simulink model "PID_ControlSim"  (R2018a)
settings: Solver=VariableStepAuto  StartTime=0.0  StopTime=10  FixedStep=0.01  MaxStep=0.01  RelTol=1e-3
values from neighbouring files (symbols this model uses):
  b = 0.5*mp*Lp*Lr*Bp    [InvPend_PID.m]
  b2 = -0.5*mp*Lp*Lr*Bp / JT    [InvPend_PID.m]
  c = 0.25*mp^2*Lp^2*Lr*gty    [InvPend_PID.m]    (also in InvPend_Params.m = 0.0318)
  c2 = 0.25*mp^2*Lp^2*Lr*gty / JT    [InvPend_PID.m]
  d = ( Jp + 0.25*mp*Lp^2 ) * ( etag*etam*kt/Rm )    [InvPend_PID.m]    (also in InvPend_Params.m = 0.1522)
  d2 = ( Jp + 0.25*mp*Lp^2 )*( etag*etam*kt )/( JT*Rm )    [InvPend_PID.m]
  f = ( Jr + mp*Lr^2 )*Bp    [InvPend_PID.m]
  g = 0.5*mp*Lp*gty*( Jr + mp*Lr^2 )    [InvPend_PID.m]
  g2 = -( Jr + mp*Lr^2 )*Bp / JT    [InvPend_PID.m]
  h = ( 0.5*mp*Lp*Lr ) * ( etag*etam*kt/Rm )    [InvPend_PID.m]
  h2 = 0.5*mp*Lp*gty*( Jr + mp*Lr^2 ) / JT    [InvPend_PID.m]
  i2 = ( 0.5*mp*Lp*Lr )*( etag*etam*kt )/( JT*Rm )    [InvPend_PID.m]
  JT = Jp*mp*Lr^2 + Jr*Jp + 0.25*Jr*mp*Lp^2    (= 2.04748555487e-06)    [InvPend_Params.m]
  Kd = K    (= 0.465)    [InvPend_PID.m]
  Ki = zc1*zc2*K    [InvPend_PID.m]
  Kp = (zc1 + zc2)*K    [InvPend_PID.m]
  q = a + d*Kg*km    [InvPend_PID.m]
  q2 = g2 + a2 + e2    [InvPend_PID.m]
  r = e + h*Kg*km    [InvPend_PID.m]    (also in InvPend_StateSpace.m = 0.35*square(0.1*2*pi*t))
  r2 = -h2 + g2*( a2 + e2 ) - b2*( f2 + j2 )    [InvPend_PID.m]
  t2 = h2*( a2 + e2 ) - c2*( f2 + j2 )    [InvPend_PID.m]
libraries: simulink_extras x2, simulink x1
settings Model: Creator=andrewchulock  LastModifiedBy=andrewchulock

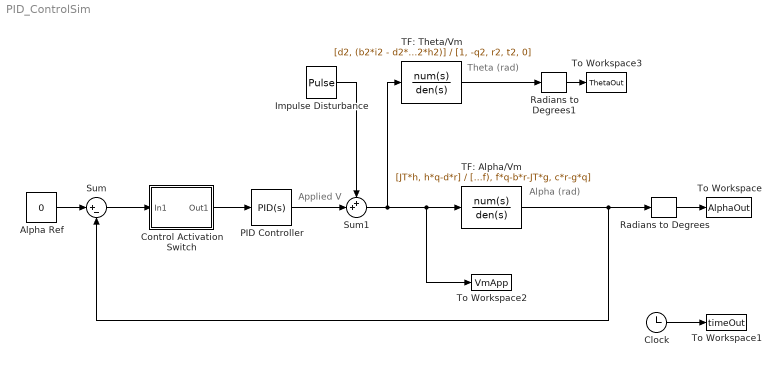
== system PID_ControlSim ==
  note: Theta (rad)
  note: Applied V
  note: Alpha (rad)
  Alpha Ref : Constant  Value=0
  Clock : Clock
  Control Activation Switch : Subsystem
  Impulse Disturbance : DiscretePulseGenerator  PulseType=Time based  Period=10  PulseWidth=0.01  PhaseDelay=1
  PID Controller : simulink/Continuous/PID Controller  Controller=PID  TimeDomain=Continuous-time  SampleTime=-1  IntegratorMethod=Forward Euler  FilterMethod=Forward Euler  Form=Parallel  UseFilter=on  ControllerParametersSource=internal  P=Kp  I=Ki  D=Kd  N=1  InitialConditionSource=internal  InitialConditionForIntegrator=0  InitialConditionForFilter=0  ExternalReset=none  LimitOutput=off  UpperSaturationLimit=inf  LowerSaturationLimit=-inf  LinearizeAsGain=on  AntiWindupMode=none  Kb=1  TrackingMode=off  Kt=1  PParamMin=[]  PParamMax=[]  IParamMin=[]  IParamMax=[]  DParamMin=[]  DParamMax=[]  NParamMin=[]  NParamMax=[]  KbParamMin=[]  KbParamMax=[]  KtParamMin=[]  KtParamMax=[]  POutMin=[]  POutMax=[]  IOutMin=[]  IOutMax=[]  DOutMin=[]  DOutMax=[]  NOutMin=[]  NOutMax=[]  KbOutMin=[]  KbOutMax=[]  KtOutMin=[]  KtOutMax=[]  IntegratorOutMin=[]  IntegratorOutMax=[]  FilterOutMin=[]  FilterOutMax=[]  SumOutMin=[]  SumOutMax=[]  SumI1OutMin=[]  SumI1OutMax=[]  SumI2OutMin=[]  SumI2OutMax=[]  SumI3OutMin=[]  SumI3OutMax=[]  SumDOutMin=[]  SumDOutMax=[]  SaturationOutMin=[]  SaturationOutMax=[]  IntegratorContinuousStateAttributes=''  IntegratorStateMustResolveToSignalObject=off  IntegratorRTWStateStorageClass=Auto  FilterContinuousStateAttributes=''  FilterStateMustResolveToSignalObject=off  FilterRTWStateStorageClass=Auto  DifferentiatorICPrevScaledInput=0  DifferentiatorOutMin=[]  DifferentiatorOutMax=[]  FilterDiffOutCoefMin=[]  FilterDiffOutCoefMax=[]  SumDenOutMin=[]  SumDenOutMax=[]  SumNumOutMin=[]  SumNumOutMax=[]  ReciprocalOutMin=[]  ReciprocalOutMax=[]  DivideOutMin=[]  DivideOutMax=[]  TunerSelectOption=Transfer Function Based (PID Tuner App)
  Radians to Degrees : simulink_extras/Transformations/Radians to Degrees
  Radians to Degrees1 : simulink_extras/Transformations/Radians to Degrees
  Sum : Sum  Inputs=|+-
  Sum1 : Sum  Inputs=++|
  TF: Alpha/Vm : TransferFcn  Numerator=[JT*h, h*q-d*r]  Denominator=[JT^2, JT*(q+f), f*q-b*r-JT*g, c*r-g*q]
  TF: Theta/Vm : TransferFcn  Numerator=[d2, (b2*i2 - d2*g2), (c2*i2 - d2*h2)]  Denominator=[1, -q2, r2, t2, 0]
  To Workspace : ToWorkspace  VariableName=AlphaOut  SampleTime=-1
      settings: Save2DSignal=2-D array (concatenate along first dimension)
  To Workspace1 : ToWorkspace  VariableName=timeOut  SampleTime=-1
      settings: Save2DSignal=2-D array (concatenate along first dimension)
  To Workspace2 : ToWorkspace  VariableName=VmApp  SampleTime=-1
      settings: Save2DSignal=2-D array (concatenate along first dimension)
  To Workspace3 : ToWorkspace  VariableName=ThetaOut  SampleTime=-1
      settings: Save2DSignal=2-D array (concatenate along first dimension)
  wires:
  TF: Alpha/Vm/1 -> Radians to Degrees/1, Sum/2
  Clock/1 -> To Workspace1/1
  Alpha Ref/1 -> Sum/1
  Control Activation Switch/1(Out1) -> PID Controller/1
  Sum/1 -> Control Activation Switch/1(In1)
  PID Controller/1 -> Sum1/2
  Sum1/1 -> TF: Theta/Vm/1, To Workspace2/1, TF: Alpha/Vm/1
  Impulse Disturbance/1 -> Sum1/1
  TF: Theta/Vm/1 -> Radians to Degrees1/1
  Radians to Degrees/1 -> To Workspace/1
  Radians to Degrees1/1 -> To Workspace3/1

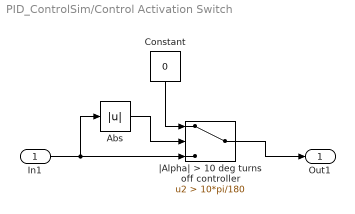
== system PID_ControlSim/Control Activation Switch ==
  In1 : Inport
  " |Alpha| > 10 deg turns off controller" : Switch  Criteria=u2 > Threshold  Threshold=10*pi/180
  Abs : Abs
  Constant : Constant  Value=0
  Out1 : Outport
  wires:
  Constant/1 -> " |Alpha| > 10 deg turns off controller"/1
  Abs/1 -> " |Alpha| > 10 deg turns off controller"/2
  " |Alpha| > 10 deg turns off controller"/1 -> Out1/1
  In1/1 -> Abs/1, " |Alpha| > 10 deg turns off controller"/3
